simulink model "block_diagram_for_induction_motor"  (R2014a)
settings: Solver=ode23t  StartTime=0.0  StopTime=3  MaxStep=1e-6  RelTol=1e-3
values from neighbouring files (symbols this model uses):
  M = input('enter modulation index: \n')    [code_for_single_phase_csi.m]    (also in code_for_single_phase_vsi.m; code_for_three_phase_csi.m; code_for_three_phase_vsi.m; code_for_vsi.m = D)
  p11 = rem(m,360)    [code_for_single_phase_csi.m]    (also in code_for_single_phase_vsi.m; code_for_three_phase_csi.m; code_for_three_phase_vsi.m; code_for_vsi.m)
  p22 = rem(n,360)    [code_for_single_phase_csi.m]    (also in code_for_single_phase_vsi.m; code_for_three_phase_csi.m; code_for_three_phase_vsi.m; code_for_vsi.m)
  p33 = rem(o,360)    [code_for_single_phase_csi.m]    (also in code_for_single_phase_vsi.m; code_for_three_phase_csi.m; code_for_three_phase_vsi.m; code_for_vsi.m)
  p44 = rem(p,360)    [code_for_single_phase_csi.m]    (also in code_for_single_phase_vsi.m; code_for_three_phase_csi.m; code_for_three_phase_vsi.m; code_for_vsi.m)
  p55 = rem(q,360)    [code_for_single_phase_csi.m]    (also in code_for_single_phase_vsi.m; code_for_three_phase_csi.m; code_for_three_phase_vsi.m; code_for_vsi.m)
  p66 = rem(r,360)    [code_for_single_phase_csi.m]    (also in code_for_single_phase_vsi.m; code_for_three_phase_csi.m; code_for_three_phase_vsi.m; code_for_vsi.m)
  p77 = rem(s,360)    [code_for_single_phase_csi.m]    (also in code_for_single_phase_vsi.m; code_for_three_phase_csi.m; code_for_three_phase_vsi.m; code_for_vsi.m)
  p88 = rem(t,360)    [code_for_three_phase_vsi.m]    (also in code_for_vsi.m)
libraries: powerlib x17, powerlib_meascontrol x2
settings Model: Creator=singa  LastModifiedBy=singa

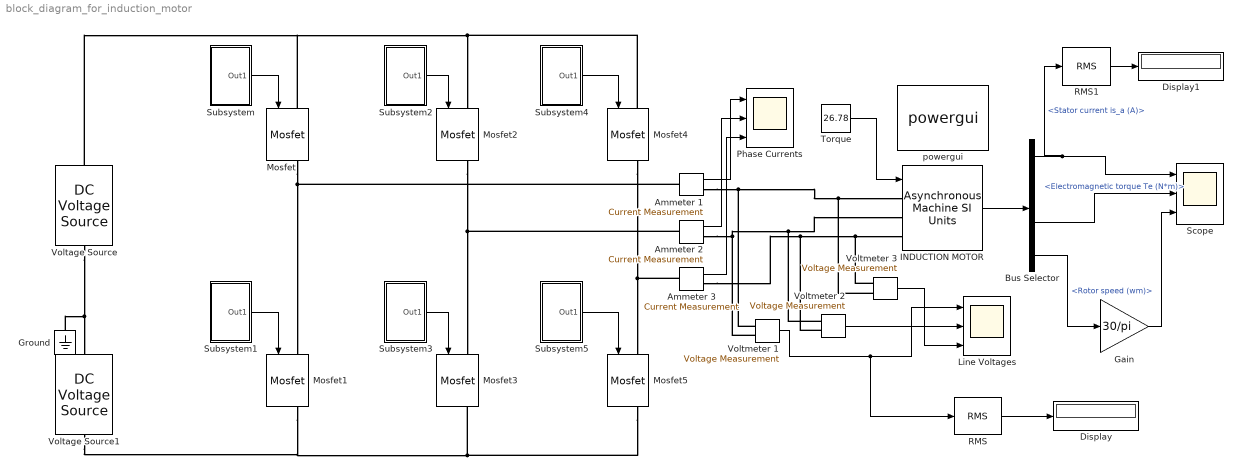
== system block_diagram_for_induction_motor ==
  Ammeter 1 : powerlib/Measurements/Current Measurement  PhasorSimulation=off  OutputType=Complex  PSBequivalent=0
  Ammeter 2 : powerlib/Measurements/Current Measurement  PhasorSimulation=off  OutputType=Complex  PSBequivalent=0
  Ammeter 3 : powerlib/Measurements/Current Measurement  PhasorSimulation=off  OutputType=Complex  PSBequivalent=0
  Bus Selector : BusSelector  OutputSignals=Stator measurements.Stator current is_a (A),Rotor measurements.Rotor current ir_a (A),Mechanical.Electromagnetic torque Te (N*m),Mechanical.Rotor speed (wm)
  Display : Display
  Display1 : Display
  Gain : Gain  Gain=30/pi
  Ground : powerlib/Elements/Ground  LConnTagsString=a
  INDUCTION MOTOR : powerlib/Machines/Asynchronous Machine SI Units  PresetModel="15:  5.4 HP (4KW)   400 V  50Hz 1430 RPM"  MechanicalLoad=Torque Tm  ShowDetailedParameters=on  RotorType=Squirrel-cage  ReferenceFrame=Rotor  Units=SI  MeasurementBus=off  NominalParameters=[4000 400 50]  Stator=[1.405 0.005839]  Rotor=[1.395 0.005839]  Cage1=[ 0.022 0.226/377]  Cage2=[ 0.022 0.226/377]  Lm=0.1722  Mechanical=[0.0131 0.002985 2]  PolePairs=2  InitialConditions=[1 0 0 0 0 0 0 0]  SimulateSaturation=off  Saturation=[14.03593122, 27.81365428, 53.79336849, 72.68890987, 97.98006896, 148.6815601, 215.7428561, 302.9841135, 420.4778367 ; 230, 322, 414, 460, 506, 552, 598, 644, 690]  LoadFlowParameters=1492000  TsPowergui=0  TsBlock=-1  IterativeModel=Trapezoidal non iterative  Pmec=0
  Line Voltages : Scope  NumInputPorts=3
      settings: YMin=-25~-500~-25  YMax=500~25~500  SampleInput=on  SampleTime=1e-6
  Mosfet{,1..5} (6 alike) : powerlib/Power Electronics/Mosfet  Ron=0.1  Lon=0  Rd=0.01  Vfd=0  IC=0  Rs=1e5  Cs=inf  Measurements=on
  Phase Currents : Scope  NumInputPorts=3
      settings: YMin=-10~-10~-9  YMax=9~10~10  SampleInput=on  SampleTime=1e-6
  RMS : powerlib_meascontrol/Measurements/RMS  TrueRMS=on  Freq=50*M  RMSInit=120  Ts=0
  RMS1 : powerlib_meascontrol/Measurements/RMS  TrueRMS=on  Freq=50*M  RMSInit=120  Ts=0
  Scope : Scope  NumInputPorts=3
      settings: YMin=-5~-5~-5  YMax=5~5~5  SaveName=ScopeData2  SampleInput=on  SampleTime=1e-6
  Subsystem : Subsystem
  Subsystem1 : Subsystem
  Subsystem2 : Subsystem
  Subsystem3 : Subsystem
  Subsystem4 : Subsystem
  Subsystem5 : Subsystem
  Torque : Constant  Value=26.78
  Voltage Source : powerlib/Electrical Sources/DC Voltage Source  Amplitude=339.5  Measurements=None
  Voltage Source1 : powerlib/Electrical Sources/DC Voltage Source  Amplitude=339.5  Measurements=None
  Voltmeter 1 : powerlib/Measurements/Voltage Measurement  PhasorSimulation=off  OutputType=Complex  PSBequivalent=0
  Voltmeter 2 : powerlib/Measurements/Voltage Measurement  PhasorSimulation=off  OutputType=Complex  PSBequivalent=0
  Voltmeter 3 : powerlib/Measurements/Voltage Measurement  PhasorSimulation=off  OutputType=Complex  PSBequivalent=0
  powergui : powerlib/powergui  Priority=1  SimulationMode=Continuous  SolverType=Tustin  SampleTime=50e-6  frequency=60  SPID=off  DisableSnubberDevices=off  DisableRonSwitches=off  DisableVfSwitches=off  SwTol=0  Interpol=off  DisplayEquations=off  Ts=0  methode=off  frequencyindice=0  Pbase=100e6  ErrMax=1e-4  Iterations=50  UnitsV=kV  UnitsW=MW  FunctionMessages=off  echomessages=off  HookPort=off  EnableUseOfTLC=off  x0status=blocks  RestoreLinks=warning  ResistiveCurrentMeasurement=off  Frange=[0:2:500]  Ylog=off  Xlog=on  ShowGrid=off  save=off  variable=ZData  structure=ScopeData2  ZoomFFT=off  StartTime=2.5  cycles=2  DisplayStyle=4  fundamental=50*1  FreqAxis=on  MaxFrequency=2500  frequencyindicesteady=1  RmsSteady=1  display=off
  wires:
  Ammeter 1/1 -> Phase Currents/1
  Ammeter 2/1 -> Phase Currents/2
  Ammeter 3/1 -> Phase Currents/3
  Torque/1 -> INDUCTION MOTOR/1
  Voltmeter 1/1 -> RMS/1, Line Voltages/1
  Voltmeter 2/1 -> Line Voltages/2
  Voltmeter 3/1 -> Line Voltages/3
  INDUCTION MOTOR/1 -> Bus Selector/1
  Bus Selector/4 -> Gain/1  "<Rotor speed (wm)>"
  Gain/1 -> Scope/3
  Bus Selector/1 -> RMS1/1, Scope/1  "<Stator current is_a (A)>"
  Subsystem/1(Out1) -> Mosfet/1
  Subsystem2/1(Out1) -> Mosfet2/1
  Subsystem4/1(Out1) -> Mosfet4/1
  Subsystem1/1(Out1) -> Mosfet1/1
  Subsystem3/1(Out1) -> Mosfet3/1
  Subsystem5/1(Out1) -> Mosfet5/1
  Bus Selector/3 -> Scope/2  "<Electromagnetic torque Te (N*m)>"
  RMS/1 -> Display/1
  RMS1/1 -> Display1/1
  connections:
  Voltage Source/LConn1 -- Voltage Source1/RConn1 -- Ground/LConn1
  Mosfet4/LConn1 -- Mosfet2/LConn1 -- Mosfet/LConn1 -- Voltage Source/RConn1
  Mosfet5/RConn1 -- Mosfet3/RConn1 -- Mosfet1/RConn1 -- Voltage Source1/LConn1
  Mosfet/RConn1 -- Ammeter 1/LConn1 -- Mosfet1/LConn1
  Mosfet2/RConn1 -- Ammeter 2/LConn1 -- Mosfet3/LConn1
  Mosfet4/RConn1 -- Ammeter 3/LConn1 -- Mosfet5/LConn1
  Ammeter 1/RConn1 -- Voltmeter 1/LConn1 -- Voltmeter 3/LConn2 -- INDUCTION MOTOR/LConn1
  Ammeter 2/RConn1 -- Voltmeter 2/LConn1 -- INDUCTION MOTOR/LConn2 -- Voltmeter 1/LConn2
  Ammeter 3/RConn1 -- Voltmeter 2/LConn2 -- Voltmeter 3/LConn1 -- INDUCTION MOTOR/LConn3

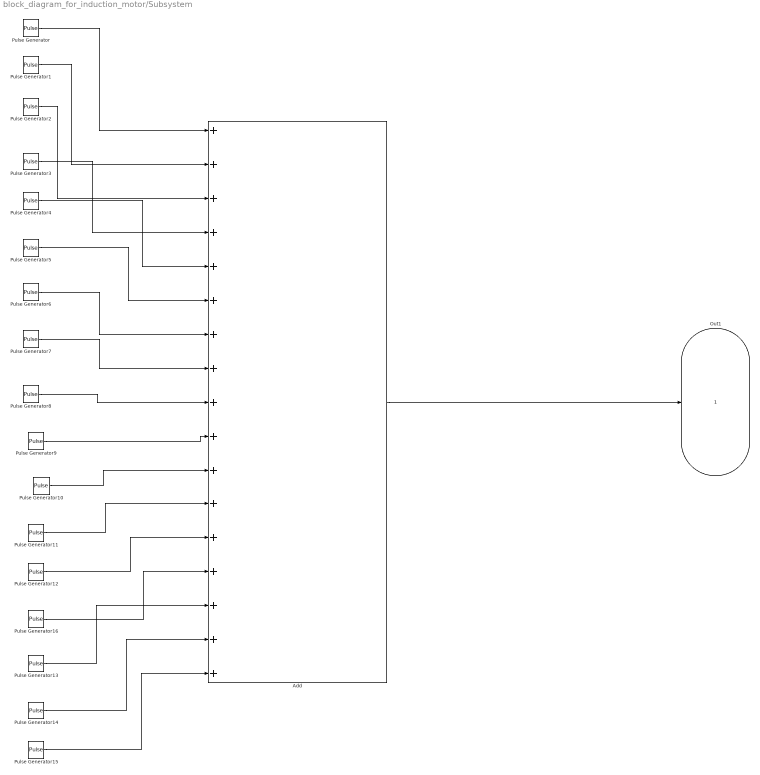
== system block_diagram_for_induction_motor/Subsystem ==
  Add : Sum  Inputs=+++++++++++++++++
  Pulse Generator : DiscretePulseGenerator  PulseType=Time based  Period=0.02/M  PulseWidth=(p11/360)*100
  Pulse Generator1 : DiscretePulseGenerator  PulseType=Time based  Period=0.02/M  PulseWidth=(p33-p22)/360*100  PhaseDelay=p22/360*0.02/M
  Pulse Generator10 : DiscretePulseGenerator  PulseType=Time based  Period=0.02/M  PulseWidth=(p44-p33)/360*100  PhaseDelay=0.01/M+p33/360*0.02/M
  Pulse Generator11 : DiscretePulseGenerator  PulseType=Time based  Period=0.02/M  PulseWidth=(p66-p55)/360*100  PhaseDelay=0.01/M+p55/360*0.02/M
  Pulse Generator12 : DiscretePulseGenerator  PulseType=Time based  Period=0.02/M  PulseWidth=(p88-p77)/360*100  PhaseDelay=0.01/M+p77/360*0.02/M
  Pulse Generator13 : DiscretePulseGenerator  PulseType=Time based  Period=0.02/M  PulseWidth=(p66-p55)/360*100  PhaseDelay=0.01/M+(180-p66)/360*0.02/M
  Pulse Generator14 : DiscretePulseGenerator  PulseType=Time based  Period=0.02/M  PulseWidth=(p44-p33)/360*100  PhaseDelay=0.01/M+(180-p44)/360*0.02/M
  Pulse Generator15 : DiscretePulseGenerator  PulseType=Time based  Period=0.02/M  PulseWidth=(p22-p11)/360*100  PhaseDelay=0.01/M+(180-p22)/360*0.02/M
  Pulse Generator16 : DiscretePulseGenerator  PulseType=Time based  Period=0.02/M  PulseWidth=(p88-p77)/360*100  PhaseDelay=0.01/M+(180-p88)/360*0.02/M
  Pulse Generator2 : DiscretePulseGenerator  PulseType=Time based  Period=0.02/M  PulseWidth=(p55-p44)/360*100  PhaseDelay=p44/360*0.02/M
  Pulse Generator3 : DiscretePulseGenerator  PulseType=Time based  Period=0.02/M  PulseWidth=(p77-p66)/360*100  PhaseDelay=p66/360*0.02/M
  Pulse Generator4 : DiscretePulseGenerator  PulseType=Time based  Period=0.02/M  PulseWidth=(90-p88)/180*100  PhaseDelay=p88/360*0.02/M
  Pulse Generator5 : DiscretePulseGenerator  PulseType=Time based  Period=0.02/M  PulseWidth=(p77-p66)/360*100  PhaseDelay=(180-p77)/360*0.02/M
  Pulse Generator6 : DiscretePulseGenerator  PulseType=Time based  Period=0.02/M  PulseWidth=(p55-p44)/360*100  PhaseDelay=(180-p55)/360*0.02/M
  Pulse Generator7 : DiscretePulseGenerator  PulseType=Time based  Period=0.02/M  PulseWidth=(p33-p22)/360*100  PhaseDelay=(180-p33)/360*0.02/M
  Pulse Generator8 : DiscretePulseGenerator  PulseType=Time based  Period=0.02/M  PulseWidth=(p11/360)*100  PhaseDelay=(180-p11)/360*0.02/M
  Pulse Generator9 : DiscretePulseGenerator  PulseType=Time based  Period=0.02/M  PulseWidth=(p22-p11)/360*100  PhaseDelay=0.01/M+p11/360*0.02/M
  Out1 : Outport
  wires:
  Pulse Generator4/1 -> Add/5
  Pulse Generator15/1 -> Add/17
  Pulse Generator6/1 -> Add/7
  Pulse Generator7/1 -> Add/8
  Pulse Generator16/1 -> Add/14
  Pulse Generator5/1 -> Add/6
  Pulse Generator9/1 -> Add/10
  Pulse Generator2/1 -> Add/3
  Pulse Generator12/1 -> Add/13
  Pulse Generator10/1 -> Add/11
  Pulse Generator11/1 -> Add/12
  Pulse Generator3/1 -> Add/4
  Pulse Generator1/1 -> Add/2
  Pulse Generator/1 -> Add/1
  Pulse Generator13/1 -> Add/15
  Pulse Generator14/1 -> Add/16
  Pulse Generator8/1 -> Add/9
  Add/1 -> Out1/1

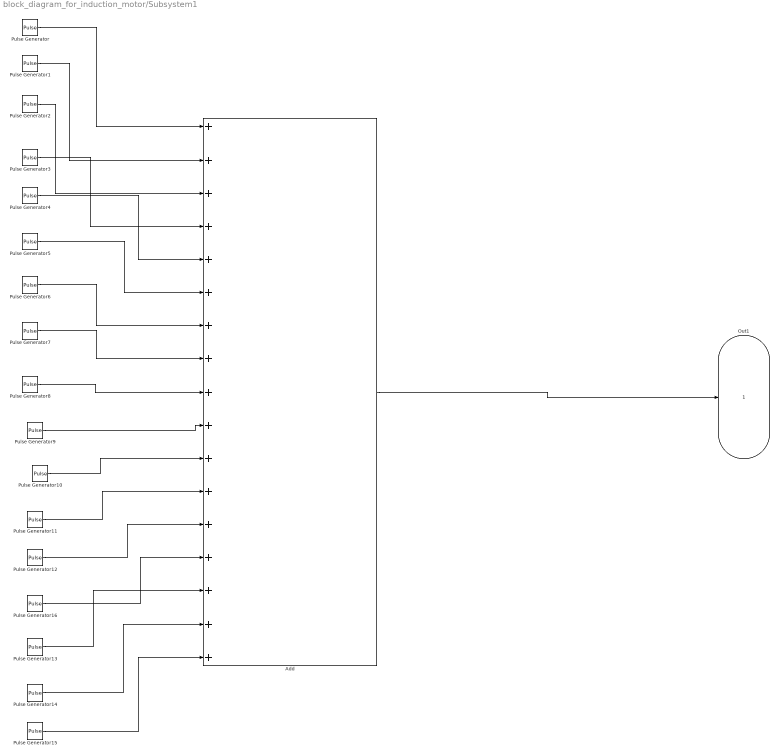
== system block_diagram_for_induction_motor/Subsystem1 ==
  Add : Sum  Inputs=+++++++++++++++++
  Pulse Generator : DiscretePulseGenerator  PulseType=Time based  Period=0.02/M  PulseWidth=(p11/360)*100  PhaseDelay=0.01/M
  Pulse Generator1 : DiscretePulseGenerator  PulseType=Time based  Period=0.02/M  PulseWidth=(p33-p22)/360*100  PhaseDelay=p22/360*0.02/M+0.01/M
  Pulse Generator10 : DiscretePulseGenerator  PulseType=Time based  Period=0.02/M  PulseWidth=(p44-p33)/360*100  PhaseDelay=0.01/M+p33/360*0.02/M+0.01/M
  Pulse Generator11 : DiscretePulseGenerator  PulseType=Time based  Period=0.02/M  PulseWidth=(p66-p55)/360*100  PhaseDelay=0.01/M+p55/360*0.02/M+0.01/M
  Pulse Generator12 : DiscretePulseGenerator  PulseType=Time based  Period=0.02/M  PulseWidth=(p88-p77)/360*100  PhaseDelay=0.01/M+p77/360*0.02/M+0.01/M
  Pulse Generator13 : DiscretePulseGenerator  PulseType=Time based  Period=0.02/M  PulseWidth=(p66-p55)/360*100  PhaseDelay=0.01/M+(180-p66)/360*0.02/M+0.01/M
  Pulse Generator14 : DiscretePulseGenerator  PulseType=Time based  Period=0.02/M  PulseWidth=(p44-p33)/360*100  PhaseDelay=0.01/M+(180-p44)/360*0.02/M+0.01/M
  Pulse Generator15 : DiscretePulseGenerator  PulseType=Time based  Period=0.02/M  PulseWidth=(p22-p11)/360*100  PhaseDelay=0.01/M+(180-p22)/360*0.02/M+0.01/M
  Pulse Generator16 : DiscretePulseGenerator  PulseType=Time based  Period=0.02/M  PulseWidth=(p88-p77)/360*100  PhaseDelay=0.01/M+(180-p88)/360*0.02/M+0.01/M
  Pulse Generator2 : DiscretePulseGenerator  PulseType=Time based  Period=0.02/M  PulseWidth=(p55-p44)/360*100  PhaseDelay=p44/360*0.02/M+0.01/M
  Pulse Generator3 : DiscretePulseGenerator  PulseType=Time based  Period=0.02/M  PulseWidth=(p77-p66)/360*100  PhaseDelay=p66/360*0.02/M+0.01/M
  Pulse Generator4 : DiscretePulseGenerator  PulseType=Time based  Period=0.02/M  PulseWidth=(90-p88)/180*100  PhaseDelay=p88/360*0.02/M+0.01/M
  Pulse Generator5 : DiscretePulseGenerator  PulseType=Time based  Period=0.02/M  PulseWidth=(p77-p66)/360*100  PhaseDelay=(180-p77)/360*0.02/M+0.01/M
  Pulse Generator6 : DiscretePulseGenerator  PulseType=Time based  Period=0.02/M  PulseWidth=(p55-p44)/360*100  PhaseDelay=(180-p55)/360*0.02/M+0.01/M
  Pulse Generator7 : DiscretePulseGenerator  PulseType=Time based  Period=0.02/M  PulseWidth=(p33-p22)/360*100  PhaseDelay=(180-p33)/360*0.02/M+0.01/M
  Pulse Generator8 : DiscretePulseGenerator  PulseType=Time based  Period=0.02/M  PulseWidth=(p11/360)*100  PhaseDelay=(180-p11)/360*0.02/M+0.01/M
  Pulse Generator9 : DiscretePulseGenerator  PulseType=Time based  Period=0.02/M  PulseWidth=(p22-p11)/360*100  PhaseDelay=0.01/M+p11/360*0.02/M+0.01/M
  Out1 : Outport
  wires:
  Pulse Generator4/1 -> Add/5
  Pulse Generator15/1 -> Add/17
  Pulse Generator6/1 -> Add/7
  Pulse Generator7/1 -> Add/8
  Pulse Generator16/1 -> Add/14
  Pulse Generator5/1 -> Add/6
  Pulse Generator9/1 -> Add/10
  Pulse Generator2/1 -> Add/3
  Pulse Generator12/1 -> Add/13
  Pulse Generator10/1 -> Add/11
  Pulse Generator11/1 -> Add/12
  Pulse Generator3/1 -> Add/4
  Pulse Generator1/1 -> Add/2
  Pulse Generator/1 -> Add/1
  Pulse Generator13/1 -> Add/15
  Pulse Generator14/1 -> Add/16
  Pulse Generator8/1 -> Add/9
  Add/1 -> Out1/1

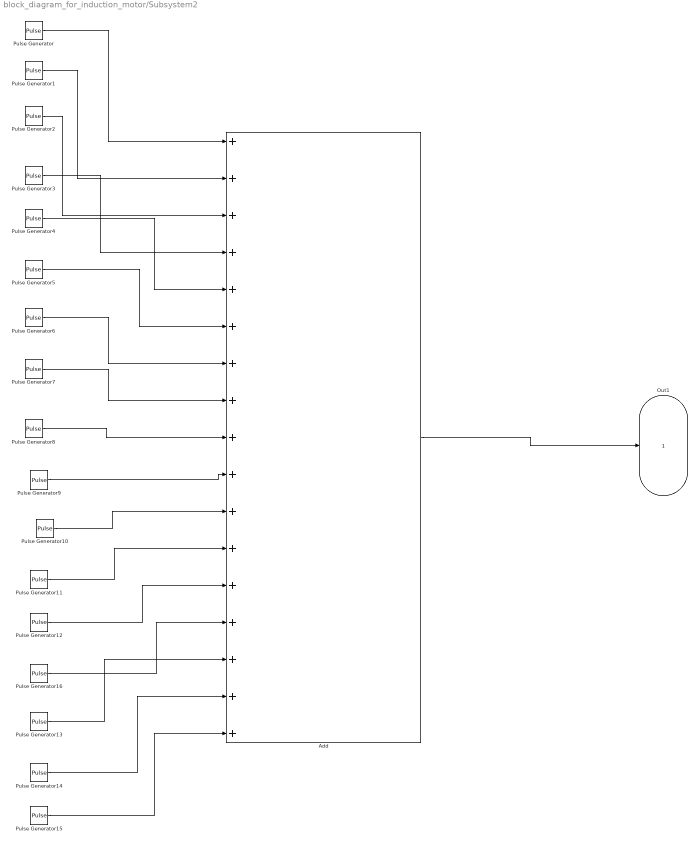
== system block_diagram_for_induction_motor/Subsystem2 ==
  Add : Sum  Inputs=+++++++++++++++++
  Pulse Generator : DiscretePulseGenerator  PulseType=Time based  Period=0.02/M  PulseWidth=(p11/360)*100  PhaseDelay=0.02/(3*M)
  Pulse Generator1 : DiscretePulseGenerator  PulseType=Time based  Period=0.02/M  PulseWidth=(p33-p22)/360*100  PhaseDelay=p22/360*0.02/M+0.02/(3*M)
  Pulse Generator10 : DiscretePulseGenerator  PulseType=Time based  Period=0.02/M  PulseWidth=(p44-p33)/360*100  PhaseDelay=0.01/M+p33/360*0.02/M+0.02/(3*M)
  Pulse Generator11 : DiscretePulseGenerator  PulseType=Time based  Period=0.02/M  PulseWidth=(p66-p55)/360*100  PhaseDelay=0.01/M+p55/360*0.02/M+0.02/(3*M)
  Pulse Generator12 : DiscretePulseGenerator  PulseType=Time based  Period=0.02/M  PulseWidth=(p88-p77)/360*100  PhaseDelay=0.01/M+p77/360*0.02/M+0.02/(3*M)
  Pulse Generator13 : DiscretePulseGenerator  PulseType=Time based  Period=0.02/M  PulseWidth=(p66-p55)/360*100  PhaseDelay=0.01/M+(180-p66)/360*0.02/M+0.02/(3*M)
  Pulse Generator14 : DiscretePulseGenerator  PulseType=Time based  Period=0.02/M  PulseWidth=(p44-p33)/360*100  PhaseDelay=0.01/M+(180-p44)/360*0.02/M+0.02/(3*M)
  Pulse Generator15 : DiscretePulseGenerator  PulseType=Time based  Period=0.02/M  PulseWidth=(p22-p11)/360*100  PhaseDelay=0.01/M+(180-p22)/360*0.02/M+0.02/(3*M)
  Pulse Generator16 : DiscretePulseGenerator  PulseType=Time based  Period=0.02/M  PulseWidth=(p88-p77)/360*100  PhaseDelay=0.01/M+(180-p88)/360*0.02/M+0.02/(3*M)
  Pulse Generator2 : DiscretePulseGenerator  PulseType=Time based  Period=0.02/M  PulseWidth=(p55-p44)/360*100  PhaseDelay=p44/360*0.02/M+0.02/(3*M)
  Pulse Generator3 : DiscretePulseGenerator  PulseType=Time based  Period=0.02/M  PulseWidth=(p77-p66)/360*100  PhaseDelay=p66/360*0.02/M+0.02/(3*M)
  Pulse Generator4 : DiscretePulseGenerator  PulseType=Time based  Period=0.02/M  PulseWidth=(90-p88)/180*100  PhaseDelay=p88/360*0.02/M+0.02/(3*M)
  Pulse Generator5 : DiscretePulseGenerator  PulseType=Time based  Period=0.02/M  PulseWidth=(p77-p66)/360*100  PhaseDelay=(180-p77)/360*0.02/M+0.02/(3*M)
  Pulse Generator6 : DiscretePulseGenerator  PulseType=Time based  Period=0.02/M  PulseWidth=(p55-p44)/360*100  PhaseDelay=(180-p55)/360*0.02/M+0.02/(3*M)
  Pulse Generator7 : DiscretePulseGenerator  PulseType=Time based  Period=0.02/M  PulseWidth=(p33-p22)/360*100  PhaseDelay=(180-p33)/360*0.02/M+0.02/(3*M)
  Pulse Generator8 : DiscretePulseGenerator  PulseType=Time based  Period=0.02/M  PulseWidth=(p11/360)*100  PhaseDelay=(180-p11)/360*0.02/M+0.02/(3*M)
  Pulse Generator9 : DiscretePulseGenerator  PulseType=Time based  Period=0.02/M  PulseWidth=(p22-p11)/360*100  PhaseDelay=0.01/M+p11/360*0.02/M+0.02/(3*M)
  Out1 : Outport
  wires:
  Pulse Generator4/1 -> Add/5
  Pulse Generator15/1 -> Add/17
  Pulse Generator6/1 -> Add/7
  Pulse Generator7/1 -> Add/8
  Pulse Generator16/1 -> Add/14
  Pulse Generator5/1 -> Add/6
  Pulse Generator9/1 -> Add/10
  Pulse Generator2/1 -> Add/3
  Pulse Generator12/1 -> Add/13
  Pulse Generator10/1 -> Add/11
  Pulse Generator11/1 -> Add/12
  Pulse Generator3/1 -> Add/4
  Pulse Generator1/1 -> Add/2
  Pulse Generator/1 -> Add/1
  Pulse Generator13/1 -> Add/15
  Pulse Generator14/1 -> Add/16
  Pulse Generator8/1 -> Add/9
  Add/1 -> Out1/1

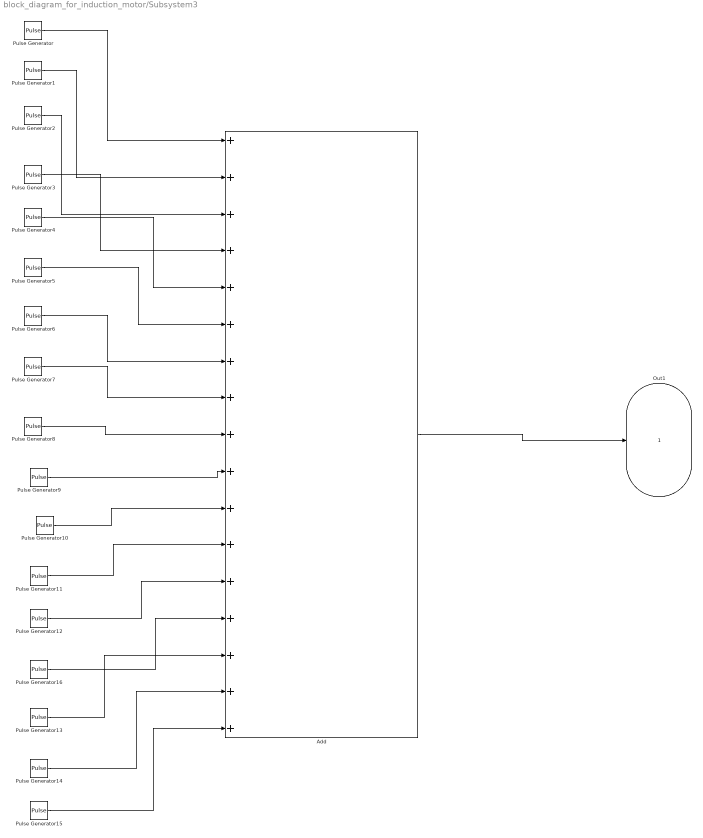
== system block_diagram_for_induction_motor/Subsystem3 ==
  Add : Sum  Inputs=+++++++++++++++++
  Pulse Generator : DiscretePulseGenerator  PulseType=Time based  Period=0.02/M  PulseWidth=(p11/360)*100  PhaseDelay=0.01/M+0.02/(3*M)
  Pulse Generator1 : DiscretePulseGenerator  PulseType=Time based  Period=0.02/M  PulseWidth=(p33-p22)/360*100  PhaseDelay=p22/360*0.02/M+0.01/M+0.02/(3*M)
  Pulse Generator10 : DiscretePulseGenerator  PulseType=Time based  Period=0.02/M  PulseWidth=(p44-p33)/360*100  PhaseDelay=0.01/M+p33/360*0.02/M+0.01/M+0.02/(3*M)
  Pulse Generator11 : DiscretePulseGenerator  PulseType=Time based  Period=0.02/M  PulseWidth=(p66-p55)/360*100  PhaseDelay=0.01/M+p55/360*0.02/M+0.01/M+0.02/(3*M)
  Pulse Generator12 : DiscretePulseGenerator  PulseType=Time based  Period=0.02/M  PulseWidth=(p88-p77)/360*100  PhaseDelay=0.01/M+p77/360*0.02/M+0.01/M+0.02/(3*M)
  Pulse Generator13 : DiscretePulseGenerator  PulseType=Time based  Period=0.02/M  PulseWidth=(p66-p55)/360*100  PhaseDelay=0.01/M+(180-p66)/360*0.02/M+0.01/M+0.02/(3*M)
  Pulse Generator14 : DiscretePulseGenerator  PulseType=Time based  Period=0.02/M  PulseWidth=(p44-p33)/360*100  PhaseDelay=0.01/M+(180-p44)/360*0.02/M+0.01/M+0.02/(3*M)
  Pulse Generator15 : DiscretePulseGenerator  PulseType=Time based  Period=0.02/M  PulseWidth=(p22-p11)/360*100  PhaseDelay=0.01/M+(180-p22)/360*0.02/M+0.01/M+0.02/(3*M)
  Pulse Generator16 : DiscretePulseGenerator  PulseType=Time based  Period=0.02/M  PulseWidth=(p88-p77)/360*100  PhaseDelay=0.01/M+(180-p88)/360*0.02/M+0.01/M+0.02/(3*M)
  Pulse Generator2 : DiscretePulseGenerator  PulseType=Time based  Period=0.02/M  PulseWidth=(p55-p44)/360*100  PhaseDelay=p44/360*0.02/M+0.01/M+0.02/(3*M)
  Pulse Generator3 : DiscretePulseGenerator  PulseType=Time based  Period=0.02/M  PulseWidth=(p77-p66)/360*100  PhaseDelay=p66/360*0.02/M+0.01/M+0.02/(3*M)
  Pulse Generator4 : DiscretePulseGenerator  PulseType=Time based  Period=0.02/M  PulseWidth=(90-p88)/180*100  PhaseDelay=p88/360*0.02/M+0.01/M+0.02/(3*M)
  Pulse Generator5 : DiscretePulseGenerator  PulseType=Time based  Period=0.02/M  PulseWidth=(p77-p66)/360*100  PhaseDelay=(180-p77)/360*0.02/M+0.01/M+0.02/(3*M)
  Pulse Generator6 : DiscretePulseGenerator  PulseType=Time based  Period=0.02/M  PulseWidth=(p55-p44)/360*100  PhaseDelay=(180-p55)/360*0.02/M+0.01/M+0.02/(3*M)
  Pulse Generator7 : DiscretePulseGenerator  PulseType=Time based  Period=0.02/M  PulseWidth=(p33-p22)/360*100  PhaseDelay=(180-p33)/360*0.02/M+0.01/M+0.02/(3*M)
  Pulse Generator8 : DiscretePulseGenerator  PulseType=Time based  Period=0.02/M  PulseWidth=(p11/360)*100  PhaseDelay=(180-p11)/360*0.02/M+0.01/M+0.02/(3*M)
  Pulse Generator9 : DiscretePulseGenerator  PulseType=Time based  Period=0.02/M  PulseWidth=(p22-p11)/360*100  PhaseDelay=0.01/M+p11/360*0.02/M+0.01/M+0.02/(3*M)
  Out1 : Outport
  wires:
  Pulse Generator4/1 -> Add/5
  Pulse Generator15/1 -> Add/17
  Pulse Generator6/1 -> Add/7
  Pulse Generator7/1 -> Add/8
  Pulse Generator16/1 -> Add/14
  Pulse Generator5/1 -> Add/6
  Pulse Generator9/1 -> Add/10
  Pulse Generator2/1 -> Add/3
  Pulse Generator12/1 -> Add/13
  Pulse Generator10/1 -> Add/11
  Pulse Generator11/1 -> Add/12
  Pulse Generator3/1 -> Add/4
  Pulse Generator1/1 -> Add/2
  Pulse Generator/1 -> Add/1
  Pulse Generator13/1 -> Add/15
  Pulse Generator14/1 -> Add/16
  Pulse Generator8/1 -> Add/9
  Add/1 -> Out1/1

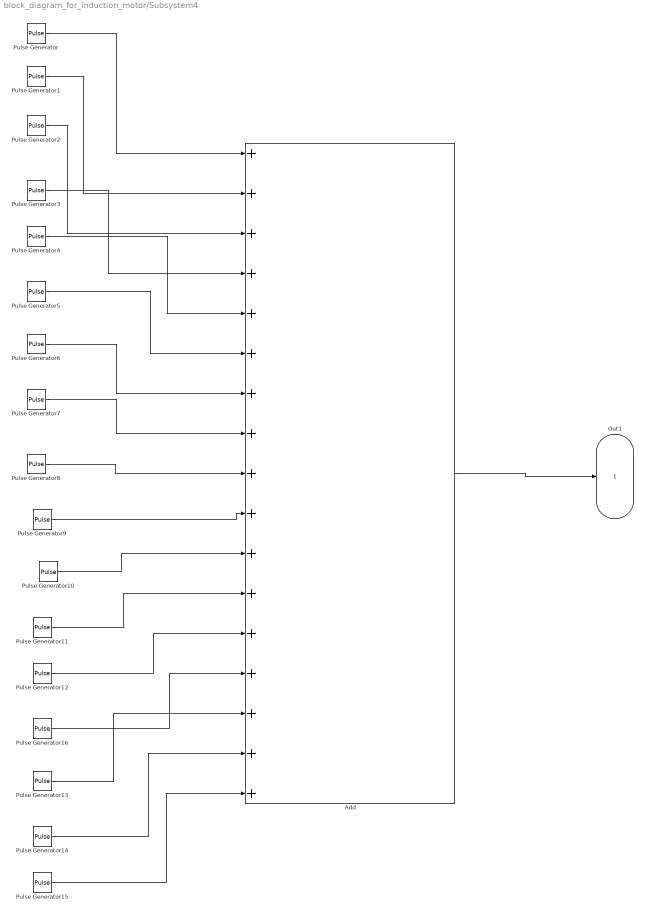
== system block_diagram_for_induction_motor/Subsystem4 ==
  Add : Sum  Inputs=+++++++++++++++++
  Pulse Generator : DiscretePulseGenerator  PulseType=Time based  Period=0.02/M  PulseWidth=(p11/360)*100  PhaseDelay=0.04/(3*M)
  Pulse Generator1 : DiscretePulseGenerator  PulseType=Time based  Period=0.02/M  PulseWidth=(p33-p22)/360*100  PhaseDelay=p22/360*0.02/M+0.04/(3*M)
  Pulse Generator10 : DiscretePulseGenerator  PulseType=Time based  Period=0.02/M  PulseWidth=(p44-p33)/360*100  PhaseDelay=0.01/M+p33/360*0.02/M+0.04/(3*M)
  Pulse Generator11 : DiscretePulseGenerator  PulseType=Time based  Period=0.02/M  PulseWidth=(p66-p55)/360*100  PhaseDelay=0.01/M+p55/360*0.02/M+0.04/(3*M)
  Pulse Generator12 : DiscretePulseGenerator  PulseType=Time based  Period=0.02/M  PulseWidth=(p88-p77)/360*100  PhaseDelay=0.01/M+p77/360*0.02/M+0.04/(3*M)
  Pulse Generator13 : DiscretePulseGenerator  PulseType=Time based  Period=0.02/M  PulseWidth=(p66-p55)/360*100  PhaseDelay=0.01/M+(180-p66)/360*0.02/M+0.04/(3*M)
  Pulse Generator14 : DiscretePulseGenerator  PulseType=Time based  Period=0.02/M  PulseWidth=(p44-p33)/360*100  PhaseDelay=0.01/M+(180-p44)/360*0.02/M+0.04/(3*M)
  Pulse Generator15 : DiscretePulseGenerator  PulseType=Time based  Period=0.02/M  PulseWidth=(p22-p11)/360*100  PhaseDelay=0.01/M+(180-p22)/360*0.02/M+0.04/(3*M)
  Pulse Generator16 : DiscretePulseGenerator  PulseType=Time based  Period=0.02/M  PulseWidth=(p88-p77)/360*100  PhaseDelay=0.01/M+(180-p88)/360*0.02/M+0.04/(3*M)
  Pulse Generator2 : DiscretePulseGenerator  PulseType=Time based  Period=0.02/M  PulseWidth=(p55-p44)/360*100  PhaseDelay=p44/360*0.02/M+0.04/(3*M)
  Pulse Generator3 : DiscretePulseGenerator  PulseType=Time based  Period=0.02/M  PulseWidth=(p77-p66)/360*100  PhaseDelay=p66/360*0.02/M+0.04/(3*M)
  Pulse Generator4 : DiscretePulseGenerator  PulseType=Time based  Period=0.02/M  PulseWidth=(90-p88)/180*100  PhaseDelay=p88/360*0.02/M+0.04/(3*M)
  Pulse Generator5 : DiscretePulseGenerator  PulseType=Time based  Period=0.02/M  PulseWidth=(p77-p66)/360*100  PhaseDelay=(180-p77)/360*0.02/M+0.04/(3*M)
  Pulse Generator6 : DiscretePulseGenerator  PulseType=Time based  Period=0.02/M  PulseWidth=(p55-p44)/360*100  PhaseDelay=(180-p55)/360*0.02/M+0.04/(3*M)
  Pulse Generator7 : DiscretePulseGenerator  PulseType=Time based  Period=0.02/M  PulseWidth=(p33-p22)/360*100  PhaseDelay=(180-p33)/360*0.02/M+0.04/(3*M)
  Pulse Generator8 : DiscretePulseGenerator  PulseType=Time based  Period=0.02/M  PulseWidth=(p11/360)*100  PhaseDelay=(180-p11)/360*0.02/M+0.04/(3*M)
  Pulse Generator9 : DiscretePulseGenerator  PulseType=Time based  Period=0.02/M  PulseWidth=(p22-p11)/360*100  PhaseDelay=0.01/M+p11/360*0.02/M+0.04/(3*M)
  Out1 : Outport
  wires:
  Pulse Generator4/1 -> Add/5
  Pulse Generator15/1 -> Add/17
  Pulse Generator6/1 -> Add/7
  Pulse Generator7/1 -> Add/8
  Pulse Generator16/1 -> Add/14
  Pulse Generator5/1 -> Add/6
  Pulse Generator9/1 -> Add/10
  Pulse Generator2/1 -> Add/3
  Pulse Generator12/1 -> Add/13
  Pulse Generator10/1 -> Add/11
  Pulse Generator11/1 -> Add/12
  Pulse Generator3/1 -> Add/4
  Pulse Generator1/1 -> Add/2
  Pulse Generator/1 -> Add/1
  Pulse Generator13/1 -> Add/15
  Pulse Generator14/1 -> Add/16
  Pulse Generator8/1 -> Add/9
  Add/1 -> Out1/1

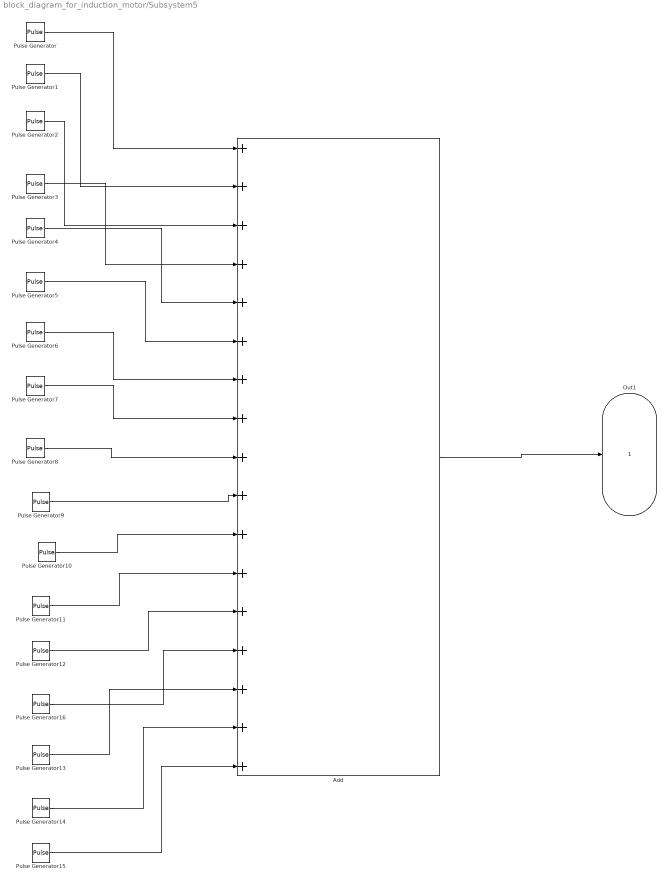
== system block_diagram_for_induction_motor/Subsystem5 ==
  Add : Sum  Inputs=+++++++++++++++++
  Pulse Generator : DiscretePulseGenerator  PulseType=Time based  Period=0.02/M  PulseWidth=(p11/360)*100  PhaseDelay=0.01/M+0.04/(3*M)
  Pulse Generator1 : DiscretePulseGenerator  PulseType=Time based  Period=0.02/M  PulseWidth=(p33-p22)/360*100  PhaseDelay=p22/360*0.02/M+0.01/M+0.04/(3*M)
  Pulse Generator10 : DiscretePulseGenerator  PulseType=Time based  Period=0.02/M  PulseWidth=(p44-p33)/360*100  PhaseDelay=0.01/M+p33/360*0.02/M+0.01/M+0.04/(3*M)
  Pulse Generator11 : DiscretePulseGenerator  PulseType=Time based  Period=0.02/M  PulseWidth=(p66-p55)/360*100  PhaseDelay=0.01/M+p55/360*0.02/M+0.01/M+0.04/(3*M)
  Pulse Generator12 : DiscretePulseGenerator  PulseType=Time based  Period=0.02/M  PulseWidth=(p88-p77)/360*100  PhaseDelay=0.01/M+p77/360*0.02/M+0.01/M+0.04/(3*M)
  Pulse Generator13 : DiscretePulseGenerator  PulseType=Time based  Period=0.02/M  PulseWidth=(p66-p55)/360*100  PhaseDelay=0.01/M+(180-p66)/360*0.02/M+0.01/M+0.04/(3*M)
  Pulse Generator14 : DiscretePulseGenerator  PulseType=Time based  Period=0.02/M  PulseWidth=(p44-p33)/360*100  PhaseDelay=0.01/M+(180-p44)/360*0.02/M+0.01/M+0.04/(3*M)
  Pulse Generator15 : DiscretePulseGenerator  PulseType=Time based  Period=0.02/M  PulseWidth=(p22-p11)/360*100  PhaseDelay=0.01/M+(180-p22)/360*0.02/M+0.01/M+0.04/(3*M)
  Pulse Generator16 : DiscretePulseGenerator  PulseType=Time based  Period=0.02/M  PulseWidth=(p88-p77)/360*100  PhaseDelay=0.01/M+(180-p88)/360*0.02/M+0.01/M+0.04/(3*M)
  Pulse Generator2 : DiscretePulseGenerator  PulseType=Time based  Period=0.02/M  PulseWidth=(p55-p44)/360*100  PhaseDelay=p44/360*0.02/M+0.01/M+0.04/(3*M)
  Pulse Generator3 : DiscretePulseGenerator  PulseType=Time based  Period=0.02/M  PulseWidth=(p77-p66)/360*100  PhaseDelay=p66/360*0.02/M+0.01/M+0.04/(3*M)
  Pulse Generator4 : DiscretePulseGenerator  PulseType=Time based  Period=0.02/M  PulseWidth=(90-p88)/180*100  PhaseDelay=p88/360*0.02/M+0.01/M+0.04/(3*M)
  Pulse Generator5 : DiscretePulseGenerator  PulseType=Time based  Period=0.02/M  PulseWidth=(p77-p66)/360*100  PhaseDelay=(180-p77)/360*0.02/M+0.01/M+0.04/(3*M)
  Pulse Generator6 : DiscretePulseGenerator  PulseType=Time based  Period=0.02/M  PulseWidth=(p55-p44)/360*100  PhaseDelay=(180-p55)/360*0.02/M+0.01/M+0.04/(3*M)
  Pulse Generator7 : DiscretePulseGenerator  PulseType=Time based  Period=0.02/M  PulseWidth=(p33-p22)/360*100  PhaseDelay=(180-p33)/360*0.02/M+0.01/M+0.04/(3*M)
  Pulse Generator8 : DiscretePulseGenerator  PulseType=Time based  Period=0.02/M  PulseWidth=(p11/360)*100  PhaseDelay=(180-p11)/360*0.02/M+0.01/M+0.04/(3*M)
  Pulse Generator9 : DiscretePulseGenerator  PulseType=Time based  Period=0.02/M  PulseWidth=(p22-p11)/360*100  PhaseDelay=0.01/M+p11/360*0.02/M+0.01/M+0.04/(3*M)
  Out1 : Outport
  wires:
  Pulse Generator4/1 -> Add/5
  Pulse Generator15/1 -> Add/17
  Pulse Generator6/1 -> Add/7
  Pulse Generator7/1 -> Add/8
  Pulse Generator16/1 -> Add/14
  Pulse Generator5/1 -> Add/6
  Pulse Generator9/1 -> Add/10
  Pulse Generator2/1 -> Add/3
  Pulse Generator12/1 -> Add/13
  Pulse Generator10/1 -> Add/11
  Pulse Generator11/1 -> Add/12
  Pulse Generator3/1 -> Add/4
  Pulse Generator1/1 -> Add/2
  Pulse Generator/1 -> Add/1
  Pulse Generator13/1 -> Add/15
  Pulse Generator14/1 -> Add/16
  Pulse Generator8/1 -> Add/9
  Add/1 -> Out1/1
